simulink model "gm_NewSignalGenerator"  (R2026a)
settings: Solver=VariableStepAuto  StopTime=5e-4
undefined symbols (not defined in the file or in its folder): ImTable, RealTable
libraries: hdlsllib x1, dsphdlxfrm2 x1
settings Model: Creator=adams
settings OptimizationCC: ConditionallyExecuteInputs=off
settings DebuggingCC: InheritedTsInSrcMsg=none

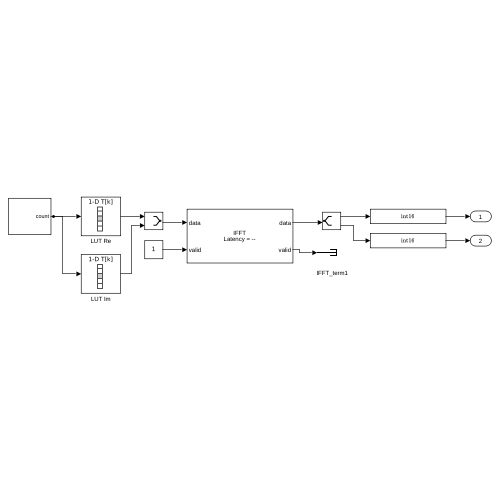
[thumbnail: Simulink's stored preview of the top-level diagram]
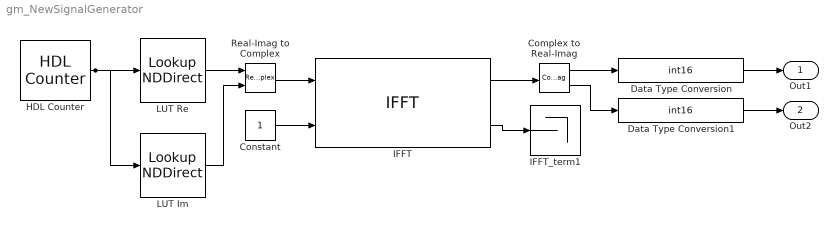
== system gm_NewSignalGenerator ==
  Complex to Real-Imag : ComplexToRealImag
  Constant : Constant  OutDataTypeStr=boolean
  Data Type Conversion : DataTypeConversion  OutDataTypeStr=int16  SaturateOnIntegerOverflow=off  RndMeth=Floor
  Data Type Conversion1 : DataTypeConversion  OutDataTypeStr=int16  SaturateOnIntegerOverflow=off  RndMeth=Floor
  HDL Counter : hdlsllib/Sources/HDL Counter  CountType=Count limited  CountInit=0  CountStep=1  CountMax=511  CountFromType=Initial value  CountFrom=0  CountResetPort=off  CountLoadPort=off  CountEnbPort=off  CountDirPort=off  CountHitOutputPort=off  CountDataType=Unsigned  CountWordLen=9  CountFracLen=0  CountSampTime=4/614400000
  IFFT : dsphdlxfrm2/IFFT  Architecture=Streaming Radix 2^2  FFTLengthSource=Property  FFTLength=512  FFTLengthMax=1024  ComplexMultiplication=Use 4 multipliers and 2 adders  BitReversedOutput=off  BitReversedInput=off  Normalize=off  SimulateUsing=Code generation  RoundingMethod=Floor  ResetInputPort=off  StartOutputPort=off  EndOutputPort=off
  IFFT_term1 : Terminator
  LUT Im : LookupNDDirect  NumberOfTableDimensions=1  Table=ImTable  TableDataTypeStr=fixdt(1,32,20)
  LUT Re : LookupNDDirect  NumberOfTableDimensions=1  Table=RealTable  TableDataTypeStr=fixdt(1,32,20)
  Real-Imag to Complex : RealImagToComplex
  Out1 : Outport  SampleTime=6.51041666666667e-09
  Out2 : Outport  Port=2  SampleTime=6.51041666666667e-09
  wires:
  Data Type Conversion1/1 -> Out2/1
  IFFT/2 -> IFFT_term1/1
  Data Type Conversion/1 -> Out1/1
  Complex to Real-Imag/2 -> Data Type Conversion1/1
  Complex to Real-Imag/1 -> Data Type Conversion/1
  IFFT/1 -> Complex to Real-Imag/1
  Constant/1 -> IFFT/2
  Real-Imag to Complex/1 -> IFFT/1
  LUT Im/1 -> Real-Imag to Complex/2
  LUT Re/1 -> Real-Imag to Complex/1
  HDL Counter/1 -> LUT Im/1, LUT Re/1
